simulink model "Throttle_dyno"  (R2022b)
settings: Solver=FixedStepAuto  StartTime=0.0  StopTime=1000  FixedStep=.01  RelTol=1e-3  EnableMultiTasking=on
libraries: canmsglib x2, raspberrypiCommlib x2
settings Model: Creator=david  LastModifiedBy=david
settings SolverCC: PositivePriorityOrder=on
settings OptimizationCC: EnhancedBackFolding=on  PassReuseOutputArgsAs=Individual arguments  ZeroExternalMemoryAtStartup=off  ZeroInternalMemoryAtStartup=off  MaxStackSize=64  OptimizeBlockOrder=speed  DifferentSizesBufferReuse=on  OptimizationCustomize=off  EfficientTunableParamExpr=on
settings DebuggingCC: ParameterTunabilityLossMsg=error
settings HardwareCC: ProdBitPerPointer=32  ProdBitPerSizeT=32  ProdBitPerPtrDiffT=32  ProdLargestAtomicInteger=Long  ProdLargestAtomicFloat=Double  ProdWordSize=32  ProdLongLongMode=on  ProdHWDeviceType=ARM Compatible->ARM Cortex
settings RTWCC: Description=Embedded Coder  SystemTargetFile=ert.tlc  HardwareBoard=Raspberry Pi  TLCOptions="-aInlineSetEventsForThisBaseRateFcn=TLC_FALSE -aSuppressMultiTaskScheduler=TLC_FALSE  -aRateBasedStepFcn=0"  TemplateMakefile=ert_default_tmf  Toolchain=GNU GCC Embedded Linux  BuildConfiguration=Faster Runs
settings CodeAppCC: ForceParamTrailComments=on  IgnoreCustomStorageClasses=off  OperatorAnnotations=on  SimulinkDataObjDesc=on  SFDataObjDesc=on  InsertBlockDesc=on
settings ERTTargetCC: SupportVariableSizeSignals=on  ExtModeTransport=2  ExtModeStaticAlloc=on  ExtModeMexFile=ext_xcp  ExtModeIntrfLevel=Level2 - Open

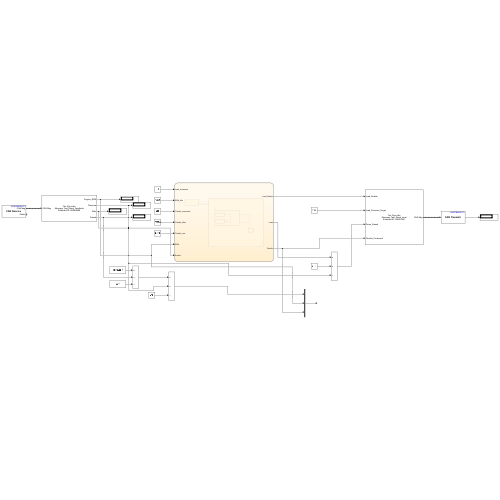
[thumbnail: Simulink's stored preview of the top-level diagram]
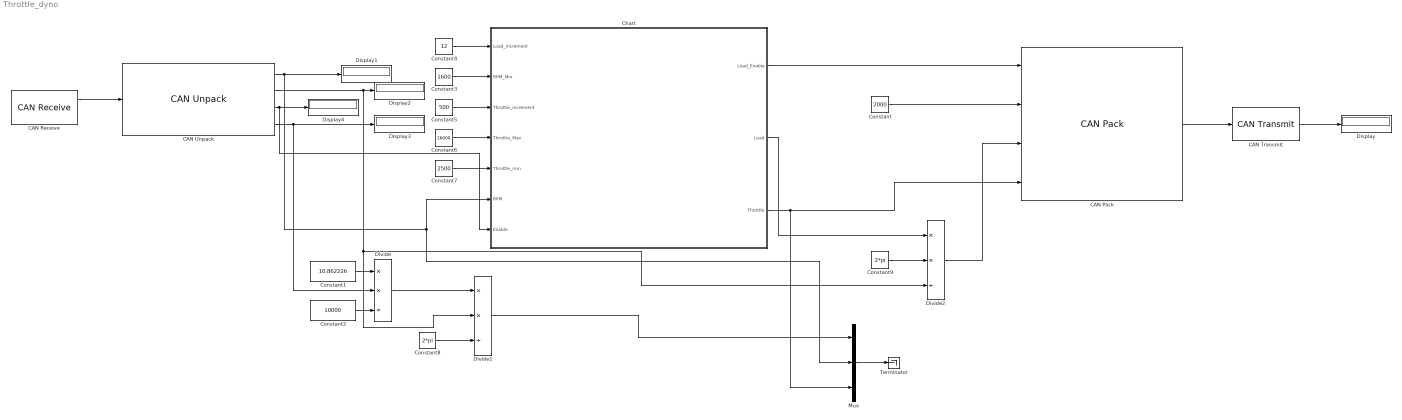
== system Throttle_dyno ==
  CAN Pack : canmsglib/CAN Pack  CANdbFile=C:\Git\2023_Tractor_Plant_Models\Dyno.dbc  MsgList=Test_Stand_Load  MsgName=Test_Stand_Load  MsgIDType=Extended (29-bit identifier)  MsgIdentifier=469827841  MsgLength=8  Remote=off  ApplyMinMax=off  BusOutput=on  SignalInfo={'Load_Enable','63','1','LE','unsigned','Standard','0','1','0','0','1';'Load_Pressure_Target','0','16','LE','unsigned','Standard','0','1','0','0','3500';'Pump_Swash','16','16','LE','unsigned','Standard','0','1','0','0','10000';'Throttle_Command','40','16','LE','unsigned','Standard','0','1','0','0','26000'}
      settings: LibrarySourceBlock=embeddedtargetslib/Host Communication/CAN Pack  DataFormat=CANdb specified signals
  CAN Receive : raspberrypiCommlib/CAN Receive  DeviceID=can0  SetupCAN=off  TypeofCAN=Real  OutputDataType=CAN Msg  IdentifierType=Standard (11-bit identifier)  MessageId=100  MsgLength=8  SampleTime=-1  OutputError=off  OutputRemote=off  SimulateUsing=Code generation
  CAN Transmit : raspberrypiCommlib/CAN Transmit  DeviceID=can0  SetupCAN=on  TypeofCAN=Real  InputDataType=CAN Msg  BlockingMode_=off  BlockTimeout_=1  OutputStatus=on  IdentifierType=Standard (11-bit identifier)  MessageId=100  MsgLength=8  RemoteFrame=off  SimulateUsing=Code generation
  CAN Unpack : canmsglib/CAN Unpack  CANdbFile=C:\Git\2023_Tractor_Plant_Models\Dyno.dbc  MsgList=Test_Stand_Feedback  MsgName=Test_Stand_Feedback  MsgIDType=Extended (29-bit identifier)  MsgIdentifier=469828098  MsgLength=8  SignalInfo={'Engine_RPM','0','16','LE','unsigned','Standard','0','1','0','0','3800';'Pressure','16','16','LE','unsigned','Standard','0','1','0','0','5000';'Start','48','1','LE','unsigned','Standard','0','1','0','0','1';'Swash','32','16','LE','unsigned','Standard','0','1','0','0','10000'}  IDPort=off  TimestampPort=off  ErrorPort=off  RemotePort=off  LengthPort=off  StatusPort=off  ApplyMinMax=off
      settings: LibrarySourceBlock=embeddedtargetslib/Host Communication/CAN Unpack  DataFormat=CANdb specified signals
  Chart : Stateflow chart  TreatAsAtomicUnit=on
  Constant : Constant  Value=2000
  Constant1 : Constant  Value=10.862226
  Constant2 : Constant  Value=10000
  Constant3 : Constant  Value=1600
  Constant4 : Constant  Value=12
  Constant5 : Constant  Value=500
  Constant6 : Constant  Value=26000
  Constant7 : Constant  Value=2500
  Constant8 : Constant  Value=2*pi
  Constant9 : Constant  Value=2*pi
  Display{,1..4} (5 alike) : Display
  Divide : Product  Inputs=**/
  Divide1 : Product  Inputs=**/
  Divide2 : Product  Inputs=**/
  Mux : Mux  Inputs=3
  Terminator : Terminator
  wires:
  CAN Receive/1 -> CAN Unpack/1
  CAN Pack/1 -> CAN Transmit/1
  Chart/1(Load_Enable) -> CAN Pack/1
  Chart/3(Throttle) -> Mux/3, CAN Pack/4
  Constant/1 -> CAN Pack/2
  Constant1/1 -> Divide/1
  Constant2/1 -> Divide/3
  CAN Unpack/1 -> Display1/1, Mux/2, Chart/6(RPM)
  Constant3/1 -> Chart/2(RPM_Min)
  Constant4/1 -> Chart/1(Load_Increment)
  Constant5/1 -> Chart/3(Throttle_Increment)
  Constant6/1 -> Chart/4(Throttle_Max)
  Constant7/1 -> Chart/5(Throttle_min)
  Divide/1 -> Divide1/1
  CAN Unpack/2 -> Display2/1, Divide2/3, Divide1/2
  Constant8/1 -> Divide1/3
  CAN Unpack/4 -> Display3/1, Divide/2
  Divide1/1 -> Mux/1
  Chart/2(Load) -> Divide2/1
  Constant9/1 -> Divide2/2
  Divide2/1 -> CAN Pack/3
  CAN Unpack/3 -> Display4/1, Chart/7(Enable)
  CAN Transmit/1 -> Display/1
  Mux/1 -> Terminator/1

== stateflow chart Throttle_dyno/Chart ==
  state Enabled
    state Throttle_Setting
      state Start
        en:
        Load_Enable=true;
        Load=0;
      state Load_Increase
        en:
        Load=Load+Load_Increment;
      (default) -> Start : {Count=0}
      (junction 21) -> Start : {Count=Count+1}
      (junction 20) -> (junction 21)
      Start -> Load_Increase
      (junction 17) -> Load_Increase
      (junction 14) -> (junction 17) [order 2]
      Load_Increase -> (junction 14) : after(5000,msec)
      (junction 14) -> (junction 20) [order 1] : [RPM<=RPM_Min]
    state End
      en,du:
      Throttle=Throttle_min;
      Load=0;
      Load_Enable=false;
    (default) -> Throttle_Setting
    (junction 28) -> Throttle_Setting : {Count=0}
    (junction 26) -> (junction 28) [order 2] : {Throttle=Throttle+Throttle_Increment}
    Throttle_Setting -> (junction 26) : [Count==5]
    (junction 26) -> End [order 1] : [Throttle>=Throttle_Max]
  state Disabled
    en,du:
    Load_Enable=false;
    Load=0;
    Throttle=Throttle_min;
  (default) -> Disabled
  Disabled -> Enabled : [hasChangedTo(Enable,true)]
  Enabled -> Disabled [order 1] : [~Enable]
  Enabled -> Disabled [order 2] : [RPM<1000]
  data: Load_Increment input; RPM_Min input; Throttle_Increment input; Throttle_Max input; Throttle_min input; Load_Enable output; Count local; Load output; Throttle output; RPM input; Enable input
